simulink model "dual_ctrl_DWC"  (R2020b)
settings: Solver=VariableStepAuto  StartTime=0.0  StopTime=0.3  FixedStep=t_step
values from neighbouring files (symbols this model uses):
  a1 = 0.3    [Parameters_simulation_feb.m]
  a2 = 0.3    [Parameters_simulation_feb.m]
  b1 = 0.3    [Parameters_simulation_feb.m]
  b2 = 0.3    [Parameters_simulation_feb.m]
  C1 = 1/((w_opt^2)*L1)    [Parameters_simulation_feb.m]
  C2 = 1/((w_opt^2)*L2)    [Parameters_simulation_feb.m]
  h = 0.3    [Parameters_simulation_feb.m]
  L1 = (mu0/pi)*(N1^2)*(a1*log((2*a1*b1)/(r1*(a1+sqrt(a1^2 + b1^2)))) + b1*log((2*a1*b1)/(r1*(b1+sqrt(a1^2 + b1^2)))) - 2*(a1 +b1 - sqrt(a1^2 + b1^2)) + 0.25*(a1 + b1))    [Parameters_simulation_feb.m]
  L2 = (mu0/pi)*(N2^2)*(a2*log((2*a2*b2)/(r2*(a2+sqrt(a2^2 + b2^2)))) + b2*log((2*a2*b2)/(r2*(b2+sqrt(a2^2 + b2^2)))) - 2*(a2 +b2 - sqrt(a2^2 + b2^2)) + 0.25*(a2 + b2))    [Parameters_simulation_feb.m]
  M = (mu0/(4*pi))*N1*N2*(-M1 + M2 + M3 - M4)    [Parameters_simulation_feb.m]
  mu0 = 4*pi*1e-7    (= 1.25663706144e-06)    [Parameters_simulation_feb.m]
  N1 = N1_max    (= 2500)    [Parameters_simulation_feb.m]
  R1 = rho_cu*N1*2*(a1+b1)/S1    (= 51.6)    [Parameters_simulation_feb.m]
  R2 = rho_cu*N2*2*(a2+b2)/S2    (= 51.6)    [Parameters_simulation_feb.m]
  S1 = S1 + 2.5e-7    (= 1.25e-06)    [Parameters_simulation_feb.m]
  speed = 20    [Parameters_simulation_feb.m]
undefined symbols (not defined in the file or in its folder): Cb, Ion, k, ki_1, kp_1, Lb, Lithium, R, t_step, Vs
libraries: powerlib x61, eePowerMeasurement x6, powerlib_meascontrol x3, electricdrivelib x1, simulink x1
settings Model: Creator=Chuanyue Li  LastModifiedBy=c2107789
settings DataIOCC: ReturnWorkspaceOutputs=off
settings DebuggingCC: ArithmeticOperatorsInVariantConditions=warning
settings SFSimCC: SimUseLocalCustomCode=off  CustomCodeUndefinedFunction=UseInterfaceOnly
settings RTWCC: RTWUseLocalCustomCode=off

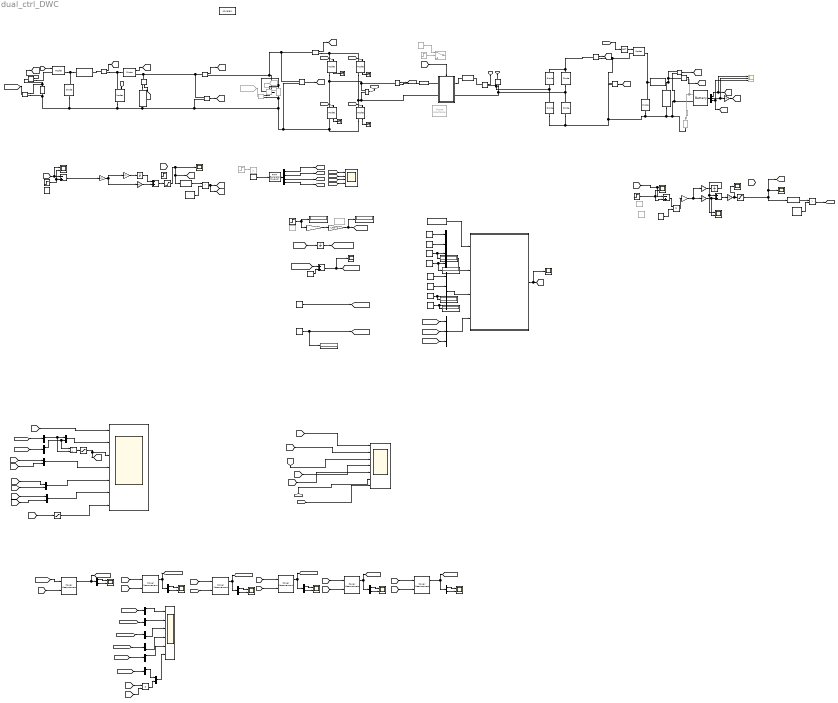
== system dual_ctrl_DWC ==
  note: Expanded implementation
  note: Inverter Control
  note: Buck-boost control
  note: Primary Coil
  note: Displacments & Airgap
  note: Velocity calc
  note: Assumed no vertical displacment
  note: Lateral (side) position
  note: Total distance moved from start
  note: assumed no side movement
  note: Height
  note: current position (relative to start)
  note: Mutual Inductance
  note: Position in driving direction
  note: Secondary Coil
  Add : Sum
  Add3 : Sum
  Add4 : Sum  Inputs=-+
  Add6 : Sum
  Add7 : Sum  Inputs=-+
  Battery1 : electricdrivelib/Extra Sources/Battery  BatType=Lithium-Ion  ShowTempParam=off  ThermalPreset=no  ShowAgeParam=off  NomV=400  NomQ=230  SOC=50  Batt_Tr=30  PresetModel=on  MaxQ=230  MinV=300  FullV=465.5949  Dis_rate=100  R=0.017391  Normal_OP=208  expZone="[432.1543          11.3]"  current=[6.5 13 32.5]  Units=Time  Tci=20  NomT=20  T2=-30  MaxQ2=4.8  FullV2=7.1  Normal_OP2=5.655  expZone2="[6.58           1]"  Rca=0.6  ti=2000  Dp=0  Neq0=0  Tsim=1e6  Ta1=25  Qeol=5.4*0.9  Reol=0.013333*1.2  Char_age=[2.3478, 3]  Dis_age=[2.3478, 10]  N1=1500  N2=10500  N3=1000  N4=1400  Ta2=45  N5=950
  Bus Creator{,1..3} (4 alike) : BusCreator  Inputs=2
  Bus Selector1 : BusSelector  OutputSignals=SOC (%),Current (A),Voltage (V)
  Constant : Constant  Value=0
  Constant1 : Constant  Value=h
  Constant2 : Constant  Value=40
  Constant3 : Constant  Commented=on  Value=10
  Constant4 : Constant
  Cp 1 : powerlib/Elements/Series RLC Branch  LConnTagsString=__new0  RConnTagsString=__new0  BranchType=C  Resistance=R  Inductance=1e-3  SetiL0=off  InitialCurrent=0  Capacitance=C1  Setx0=off  InitialVoltage=0  Measurements=None
  Cs 1 : powerlib/Elements/Series RLC Branch  LConnTagsString=__new0  RConnTagsString=__new0  BranchType=C  Resistance=R  Inductance=1e-3  SetiL0=off  InitialCurrent=0  Capacitance=C2  Setx0=off  InitialVoltage=0  Measurements=None
  Current Measurement{,1..3,7} (5 alike) : powerlib/Measurements/Current Measurement  PhasorSimulation=off  OutputType=Complex  PSBequivalent=0
  Current Measurement4 : powerlib/Measurements/Current Measurement  Commented=on  PhasorSimulation=off  OutputType=Complex  PSBequivalent=0
  DC Voltage Source : powerlib/Electrical Sources/DC Voltage Source  Amplitude=Vs  Measurements=None
  DC Voltage Source1 : powerlib/Electrical Sources/DC Voltage Source  Commented=on  Amplitude=Vs  Measurements=None
  DC Voltage Source2 : powerlib/Electrical Sources/DC Voltage Source  Commented=on  Amplitude=430  Measurements=None
  Demux : Demux
  Demux{1..14} (14 alike) : Demux  Outputs=2
  Diode : powerlib/Power Electronics/Diode  Ron=0.001  Lon=0  Vf=0  IC=0  UseSnubber=0  Rs=500000  Cs=250e-9  Measurements=on
  Diode1 : powerlib/Power Electronics/Diode  Ron=0.001  Lon=0  Vf=0.8  IC=0  UseSnubber=0  Rs=500  Cs=250e-9  Measurements=on
  Diode11 : powerlib/Power Electronics/Diode  Ron=0.001  Lon=0  Vf=0  IC=0  UseSnubber=0  Rs=500000  Cs=250e-9  Measurements=on
  Diode{2..4,7} (4 alike) : powerlib/Power Electronics/Diode  Ron=0.001  Lon=0  Vf=0.8  IC=0  UseSnubber=0  Rs=500  Cs=250e-9  Measurements=off
  Display{,1..3,5..7} (7 alike) : Display
  Divide : Product  Inputs=*/  OutMin=[0]  OutMax=[1]
  Fcn : Fcn  Expr=u(1)*2-1
  Fcn2 : Fcn  Expr=u(1)*2-1
  Gain : Gain  Gain=-1
  Gain10 : Gain  Gain=ki_1*10
  Gain11 : Gain  Gain=kp_1*10
  Gain12 : Gain  Gain=-1
  Gain13 : Gain  Gain=1e3
  Gain14 : Gain
  Gain5 : Gain  Gain=1/10
  Gain8 : Gain  Gain=k*0+1/100
  Goto18 : Goto  Commented=on  GotoTag=isource
  Goto26 : Goto  Commented=on  GotoTag=vsource
  I{2..3,8..9} (4 alike) : powerlib/Measurements/Current Measurement  PhasorSimulation=off  OutputType=Complex  PSBequivalent=0
  Initial_position : Constant  Value=-0.5
  Integrator : Integrator
  Integrator2 : Integrator  LimitOutput=on  UpperSaturationLimit=0  LowerSaturationLimit=-1
  Integrator3 : Integrator  InitialCondition=0.6
  MPH : Constant  Commented=on  Value=60
  Miles to m : Gain  Gain=1e3*1.609
  Mosfet : powerlib/Power Electronics/Mosfet  Ron=0.01  Lon=0  Rd=0.01  Vfd=0  IC=0  Rs=1e5  Cs=inf  Measurements=on
  Mosfet1 : powerlib/Power Electronics/Mosfet  Ron=0.01  Lon=0  Rd=0.01  Vfd=0  IC=0  Rs=1e5  Cs=inf  Measurements=on
  Mutual Inductance : powerlib/Elements/Mutual Inductance  Commented=on  LConnTagsString=a|b  RConnTagsString=A|B  TypeOfMutual=Two or three windings with equal mutual terms  NumberOfWindings=3  SelfImpedance1=[R1 L1]  SelfImpedance2=[R2 L2]  ThreeWindings=off  SelfImpedance3=[ 1.1 1.1e-03]  MutualImpedance=[0 M]  InductanceMatrix="[1.0 0.9  0.9 ;  0.9 1.0  0.9;  0.9 0.9 1.0 ] * 1e-3"  ResistanceMatrix="[1.0 0.9  0.9 ;  0.9 1.0  0.9;  0.9 0.9 1.0 ]"  Measurements=None
      settings: AttributesFormatString=\n  SourceProductBaseCode=PS
  Mutual_inductace_calculation : MATLAB Function  TreatAsAtomicUnit=on
  Mux : Mux  Inputs=2
  Mux1 : Mux
  Mux2 : Mux
  Mux3 : Mux  Inputs=3
  NOT : Logic  Operator=NOT  IconShape=distinctive  AllPortsSameDT=off  OutDataTypeStr=boolean
  N_primary2 : Constant  Value=N1
  N_secondary2 : Constant  Value=N1
  PWM Generator (2-Level)2 : powerlib_meascontrol/Pulse & Signal Generators/PWM Generator (2-Level)  ModulatorType=Single-phase full-bridge - Bipolar modulation (4 pulses)  ModulatorMode=Unsynchronized  Fc=f_opt  Pc=90  nF=27  MinMax="[ 0  1 ]"  SamplingTechnique=Natural  ModulatingSignals=off  m=0.8  Freq=60  Phase=0  Ts=0  ShowCarrierOutport=off
  Permiability2 : Constant  Value=mu0
  Power Measurement1 : eePowerMeasurement/Power Measurement  LabelModeActiveChoice=Continuous  F=20e3  K=[0 1]  Ts=0
      settings: SourceProductBaseCode=PS
  Power Measurement2 : eePowerMeasurement/Power Measurement  LabelModeActiveChoice=Continuous  F=s_fre  K=[0 1]  Ts=0
      settings: SourceProductBaseCode=PS
  Power Measurement{3..6} (4 alike) : eePowerMeasurement/Power Measurement  LabelModeActiveChoice=Continuous  F=f_opt  K=[0 1]  Ts=0
      settings: SourceProductBaseCode=PS
  Product : Product
  Product1 : Product  Commented=on
  Product2 : Product
  Ramp : simulink/Sources/Ramp  Commented=on  slope=200  start=0  InitialOutput=0
  Relational Operator : RelationalOperator  Operator=>  OutDataTypeStr=boolean  RndMeth=Zero
  Relational Operator2 : RelationalOperator  Operator=>  OutDataTypeStr=boolean  RndMeth=Zero
  S{3,9..12} (5 alike) : powerlib/Power Electronics/Mosfet  Ron=0.1  Lon=0  Rd=Rds  Vfd=0  IC=0  Rs=1e5  Cs=inf  Measurements=on
  S_primary2 : Constant  Value=S1
  S_secondary2 : Constant  Value=S1
  Saturation : Saturate  UpperLimit=inf  LowerLimit=0
  Saturation1 : Saturate  UpperLimit=0.95  LowerLimit=-1
  Saturation3 : Saturate  UpperLimit=1  LowerLimit=0
  Saturation4 : Saturate  UpperLimit=1  LowerLimit=0
  Scope : Scope  NumInputPorts=7
  Scope{1..2,4,19,22} (5 alike) : Scope
  Scope{6..10,12..13,18,21} (9 alike) : Scope  NumInputPorts=2
  Scope11 : Scope  NumInputPorts=4
  Scope14 : Scope  NumInputPorts=6
  Scope3 : Scope  NumInputPorts=7
  Scope5 : Scope  Commented=on  NumInputPorts=3
  Series RLC Branch : powerlib/Elements/Series RLC Branch  LConnTagsString=__new0  RConnTagsString=__new0  BranchType=L  Resistance=1  Inductance=Lb  SetiL0=on  InitialCurrent=100  Capacitance=1e-6  Setx0=off  InitialVoltage=0  Measurements=None
  Series RLC Branch1 : powerlib/Elements/Series RLC Branch  LConnTagsString=__new0  RConnTagsString=__new0  BranchType=C  Resistance=1  Inductance=1e-3  SetiL0=off  InitialCurrent=0  Capacitance=Cb  Setx0=on  InitialVoltage=400  Measurements=None
  Series RLC Branch3 : powerlib/Elements/Series RLC Branch  Commented=on  LConnTagsString=__new0  RConnTagsString=__new0  BranchType=R  Resistance=0.02  Inductance=1e-3  SetiL0=off  InitialCurrent=0  Capacitance=10e-3  Setx0=on  InitialVoltage=400  Measurements=None
  Series RLC Branch5 : powerlib/Elements/Series RLC Branch  LConnTagsString=__new0  RConnTagsString=__new0  BranchType=L  Resistance=1  Inductance=50e-3  SetiL0=on  InitialCurrent=10  Capacitance=1e-6  Setx0=off  InitialVoltage=0  Measurements=None
  Series RLC Branch9 : powerlib/Elements/Series RLC Branch  LConnTagsString=__new0  RConnTagsString=__new0  BranchType=C  Resistance=1  Inductance=1e-3  SetiL0=off  InitialCurrent=0  Capacitance=10e-3  Setx0=on  InitialVoltage=400  Measurements=None
  Step : Step  Commented=on  Time=0.05  Before=0.3  After=0.35  SampleTime=0
  Step1 : Step  Time=0  After=speed*0 + 10  SampleTime=0
  Step19 : Step  Time=0.1  Before=10  After=12  SampleTime=0
  Step2 : Step  Time=0.3  Before=0.5  After=0.5  SampleTime=0
  Step3 : Step  Commented=on  Time=0.02  Before=1  After=0  SampleTime=0
  Step4 : Step  Time=0.05  Before=100  After=50  SampleTime=0
  Subsystem1 : Subsystem
      settings: PortSchema="{\"entries\":[{\"content\":{\"sides\":[{\"content\":{\"connectorIds\":[\"LConn1\",\"LConn2\"]},\"type\":\"ConnectorPlacement.EquallySpacedRectSide\",\"uuid\":\"dc2bcdb6-339b-4429-bac0-92f3c92c18cf\"},{\"content\":{\"connectorIds\":[\"RConn1\",\"RConn2\"],\"side\":\"RIGHT\"},\"type\":\"ConnectorPlacement.EquallySpacedRectSide\",\"uuid\":\"b0ad11da-e286-4d85-af23-59a8fde2f407\"},{\"content\":{\"connectorIds\":[\"In1\"],\"side\":\"TOP\"},\"type\":\"ConnectorPlacement.EquallySpacedRectSide\",\"uuid\":\"877cda52-a106-40c9-ba33-8eb6041f6ad7\"},{\"content\":{\"connectorIds\":[],\"side\":\"HIDDEN\"},\"type\":\"ConnectorPlacement.EquallySpacedRectSide\",\"uuid\":\"0e4f87e0-ec1d-4257-a5bd-1d06479f0226\"}]},\"type\":\"ConnectorPlacement.EquallySpacedConnector\",\"uuid\":\"a87b5a18-e0dc-451c-be30-4cd433b35579\"}],\"packageUris\":[\"http://schema.mathworks.com/mf0/Connector/R2020b\"],\"version\":\"1.0\"}"
  Switch : Switch  Commented=on  Criteria=u2 > Threshold
  Terminator{16..17,22..23} (4 alike) : Terminator
  Triangle Generator : powerlib_meascontrol/Pulse & Signal Generators/Triangle Generator  Freq=s_fre  Phase=0  Ts=0
  Triangle Generator2 : powerlib_meascontrol/Pulse & Signal Generators/Triangle Generator  Freq=s_fre  Phase=0  Ts=0
  V_S1 : powerlib/Measurements/Voltage Measurement  PhasorSimulation=off  OutputType=Complex  PSBequivalent=0
  V_S2 : powerlib/Measurements/Voltage Measurement  PhasorSimulation=off  OutputType=Complex  PSBequivalent=0
  V_S3 : powerlib/Measurements/Voltage Measurement  PhasorSimulation=off  OutputType=Complex  PSBequivalent=0
  V_p2 : powerlib/Measurements/Voltage Measurement  PhasorSimulation=off  OutputType=Complex  PSBequivalent=0
  Voltage Measurement : powerlib/Measurements/Voltage Measurement  PhasorSimulation=off  OutputType=Complex  PSBequivalent=0
  Voltage Measurement1 : powerlib/Measurements/Voltage Measurement  Commented=on  PhasorSimulation=off  OutputType=Complex  PSBequivalent=0
  Voltage Measurement2 : powerlib/Measurements/Voltage Measurement  PhasorSimulation=off  OutputType=Complex  PSBequivalent=0
  Voltage Measurement5 : powerlib/Measurements/Voltage Measurement  PhasorSimulation=off  OutputType=Complex  PSBequivalent=0
  Zero : Constant  Commented=on  Value=0  OutDataTypeStr=Inherit: Inherit via back propagation
  Zero1 : Constant  Value=0.5  OutDataTypeStr=Inherit: Inherit via back propagation
  a_primary1 : Constant  Value=a1
  a_secondary2 : Constant  Value=a2
  b_primary2 : Constant  Value=b1
  b_secondary2 : Constant  Value=b2
  hour to seconds : Gain  Gain=1/60^2
  ms-1 : Constant  Commented=on  Value=speed
  powergui : powerlib/powergui  Priority=1  SimulationMode=Continuous  SampleTime=t_step  frequency=60  Iterations=50  frequencyindice=0  Pbase=100e6  ErrMax=1e-4  UnitsV=kV  UnitsW=MW  buscounter=0  FunctionMessages=off  echomessages=off  EnableUseOfTLC=off  CurrentSourceSwitches=off  DisableSnubberDevices=off  DisableRonSwitches=off  DisableVfSwitches=off  DisplayEquations=off  AutomaticDiscreteSolvers=off  SolverType=Tustin/Backward Euler (TBE)  Interpol=off  ExternalGateDelay=off  methode=off  Ts=100  x0status=blocks  SPID=off  SwTol=0  HookPort=off  NonlinearTolerance=1e-4  nMaxIteration=100  ContinueOnMaxIteration=off  RestoreLinks=warning  ResistiveCurrentMeasurement=off  Frange=[0:2:500]  Ylog=off  Xlog=on  ShowGrid=off  save=off  variable=ZData  structure=logsout  ZoomFFT=off  StartTime=0.2  cycles=10  DisplayStyle=2  fundamental=50  FreqAxis=off  MaxFrequency=1000  frequencyindicesteady=1  RmsSteady=1  display=off
  wires:
  Demux/4 -> [S4]
  [S3] -> Scope11/3
  Demux/3 -> [S3]
  [S4] -> S10/1
  I8/1 -> [Ip1]
  Demux/1 -> [S1]
  [S2] -> Scope11/2
  S12/1 -> Terminator17/1
  S11/1 -> Terminator23/1
  [S4] -> Scope11/4
  S10/1 -> Terminator16/1
  Current Measurement3/1 -> [I_in]  "Input Current"
  [S2] -> S12/1
  S9/1 -> Terminator22/1
  [S3] -> S11/1
  V_p2/1 -> [V_p1]
  [S1] -> Scope11/1
  PWM Generator (2-Level)2/1 -> Demux/1
  Demux/2 -> [S2]
  V_S2/1 -> [Vs1]  "v2"
  Step/1 -> Product1/1
  [S1] -> S9/1
  I9/1 -> [Is1]  "i2"
  Zero1/1 -> PWM Generator (2-Level)2/1
  Integrator3/1 -> Add6/1
  Fcn/1 -> Relational Operator/1
  Add6/1 -> Saturation1/1
  Diode11/1 -> [iDIO]
  [s2] -> Mosfet1/1
  Current Measurement/1 -> [il]
  Current Measurement1/1 -> [io_dcdc]
  Gain10/1 -> Integrator3/1
  Current Measurement2/1 -> [ic]
  Triangle Generator/1 -> Relational Operator/2
  [s1] -> Mosfet/1
  Add7/1 -> Gain8/1
  [il] -> Scope7/1, Add7/1
  Gain8/1 -> Gain11/1, Gain10/1
  Voltage Measurement/1 -> [vc]
  Relational Operator/1 -> [s1], [s2]
  Step4/1 -> Scope7/2, Add7/2  "il_target"
  Gain11/1 -> Add6/2
  Current Measurement7/1 -> [isource]
  [isource] -> Power Measurement1/2
  Voltage Measurement5/1 -> [vsource]
  [vsource] -> Power Measurement1/1
  Power Measurement1/1 -> [input_power], Demux3/1  "Input power (source)"
  Demux3/2 -> Scope18/2
  Demux3/1 -> Scope18/1
  Gain13/1 -> Integrator2/1
  Gain5/1 -> Gain13/1, Gain14/1
  Product/1 -> Gain5/1
  Battery1/1 -> Bus Selector1/1
  Saturation4/1 -> [d_REC], Scope22/1, Fcn2/1
  Integrator2/1 -> Scope8/1, Add3/1
  Gain14/1 -> Scope8/2, Add3/2
  Bus Selector1/1 -> Scope5/1, [SOC]  "<SOC (%)>"
  Bus Selector1/3 -> [Vo_b], Scope5/3  "<Voltage (V)>"
  Gain/1 -> [Io_b]
  Fcn2/1 -> Relational Operator2/1
  Triangle Generator2/1 -> Relational Operator2/2
  Gain12/1 -> Scope19/1, Saturation4/1
  Add3/1 -> Gain12/1
  Relational Operator2/1 -> [t1]
  Step19/1 -> Add4/2, Scope21/2  "io_target"
  Bus Selector1/2 -> Scope5/2, Gain/1  "<Current (A)>"
  Saturation1/1 -> Fcn/1, [D], Scope4/1  "D1"
  [input_power] -> Demux1/1
  Bus Creator/1 -> Scope3/2  "power_comp"
  [Vo] -> Power Measurement2/1
  [Io] -> Power Measurement2/2
  Demux2/1 -> Scope6/1
  Demux2/2 -> Scope6/2
  Power Measurement2/1 -> Demux2/1, [output_power]
  [output_power] -> Demux4/1
  Demux1/1 -> Bus Creator/1, Divide/2  "input power"
  Demux4/1 -> Bus Creator/2, Divide/1  "output power"
  Saturation3/1 -> [eff], Scope3/3  "efficiency"
  Divide/1 -> Saturation3/1  "efficiency"
  [D] -> Bus Creator1/1  "praimry buck bost"
  [d_REC] -> Bus Creator1/2  "secondary rectifier"
  V_S1/1 -> [vrec]  "vrrec"
  [il] -> Bus Creator2/1  "praimry buck boost"
  [irec] -> Bus Creator2/2  "secondary rectifier output"
  Bus Creator2/1 -> Scope3/5  "inductor currents"
  [vc] -> Bus Creator3/1  "primary buck boost"
  [vrec] -> Bus Creator3/2  "secondary rectifier output"
  Bus Creator3/1 -> Scope3/6  "capcitor voltages"
  Bus Creator1/1 -> Scope3/4  "duty cycles"
  [Io] -> Saturation/1  "output current"
  [eff] -> Scope/1  "eff"
  [il] -> Scope/2  "il"
  [ic] -> Scope/3  "ic"
  [vc] -> Scope/4  "vc"
  [io_dcdc] -> Scope/5  "iodc"
  [V_p1] -> Scope/6  "vp"
  [Ip1] -> Scope/7  "Ip"
  a_primary1/1 -> Display/1, Mux1/3  "width (x)"
  Mutual_inductace_calculation/1(M) -> [M], Scope2/1
  Integrator/1 -> [displacment]
  hour to seconds/1 -> Display7/1, [speed_ms]
  Mux3/1 -> Mutual_inductace_calculation/4(displacments)
  [speed_ms] -> Integrator/1  "speed"
  Constant/1 -> [side_position]
  Step1/1 -> Display6/1, Miles to m/1
  Miles to m/1 -> hour to seconds/1
  [displacment] -> Add/1
  Mux1/1 -> Mutual_inductace_calculation/2(params_primary)  "Primary coil parameters"
  [side_position] -> Mux3/1  "x"
  S_secondary2/1 -> Mux2/2
  b_secondary2/1 -> Display3/1, Mux2/4  "height (y)"
  N_primary2/1 -> Mux1/1
  Mux2/1 -> Mutual_inductace_calculation/3(params_secondary)  "Secondary Coil Parameters"
  S_primary2/1 -> Mux1/2
  N_secondary2/1 -> Mux2/1
  [height_position] -> Mux3/3  "airgap"
  Permiability2/1 -> Mutual_inductace_calculation/1(mu)
  Add/1 -> Scope1/1, [fwd_position]  "position"
  [fwd_position] -> Mux3/2  "y"
  Initial_position/1 -> Add/2
  b_primary2/1 -> Display1/1, Mux1/4  "height (y)"
  Constant1/1 -> Display5/1, [height_position]
  a_secondary2/1 -> Display2/1, Mux2/3  "width (x)"
  Zero/1 -> Switch/1  "M"
  Step3/1 -> Switch/2
  [M] -> Subsystem1/1(M)  "M"
  [M] -> Scope3/1  "Mutual Inductance"
  Current Measurement4/1 -> Goto18/1
  Voltage Measurement1/1 -> Goto26/1
  Add4/1 -> Product/1
  Constant4/1 -> Product/2
  V_S3/1 -> [Vo]  "vcap"
  Saturation/1 -> Scope3/7  "Output Current"
  [t1] -> NOT/1
  NOT/1 -> S3/1
  I2/1 -> [Io]
  [Io] -> Add4/1, Scope21/1
  I3/1 -> [irec]
  [vrec] -> Power Measurement3/1
  [irec] -> Power Measurement3/2
  Power Measurement3/1 -> [rectifier_power], Demux5/1
  Demux5/2 -> Scope9/2
  Demux5/1 -> Scope9/1
  Demux6/1 -> Scope10/1
  Demux6/2 -> Scope10/2
  Power Measurement4/1 -> Demux6/1, [secondary_power]
  [Is1] -> Power Measurement4/2
  [Vs1] -> Power Measurement4/1
  [V_p1] -> Power Measurement5/1
  [Ip1] -> Power Measurement5/2
  Power Measurement5/1 -> [primary_power], Demux7/1
  Demux7/2 -> Scope12/2
  Demux7/1 -> Scope12/1
  Voltage Measurement2/1 -> [V_in]
  Demux8/1 -> Scope13/1
  Demux8/2 -> Scope13/2
  Power Measurement6/1 -> Demux8/1, [inv_input_power]
  [I_in] -> Power Measurement6/2
  [V_in] -> Power Measurement6/1
  [input_power] -> Demux9/1
  Demux9/1 -> Scope14/1
  [inv_input_power] -> Demux10/1
  Demux10/1 -> Scope14/2
  [primary_power] -> Demux11/1
  Demux11/2 -> Scope14/3
  Demux12/2 -> Scope14/4
  [secondary_power] -> Demux12/1
  Demux13/1 -> Scope14/5
  [rectifier_power] -> Demux13/1
  [output_power] -> Demux14/1
  Demux14/1 -> Mux/1
  Mux/1 -> Scope14/6
  Product2/1 -> Mux/2
  [Vo] -> Product2/1
  [Io] -> Product2/2
  connections:
  DC Voltage Source1/LConn1 -- Voltage Measurement1/LConn2 -- Voltage Measurement2/LConn2 -- S10/RConn1 -- S12/RConn1 -- Diode/LConn1 -- Voltage Measurement5/LConn2 -- DC Voltage Source/LConn1 -- Mosfet1/RConn1 -- Series RLC Branch1/RConn1 -- Voltage Measurement/LConn2
  V_p2/LConn2 -- Subsystem1/LConn2 -- S11/RConn1 -- S10/LConn1
  V_S2/LConn1 -- I9/RConn1 -- Diode7/RConn1 -- Diode2/LConn1
  Current Measurement3/RConn1 -- S11/LConn1 -- S9/LConn1
  V_p2/LConn1 -- S9/RConn1 -- S12/LConn1 -- I8/LConn1
  V_S2/LConn2 -- Subsystem1/RConn2 -- Diode3/RConn1 -- Diode4/LConn1
  I8/RConn1 -- Cp 1/RConn1
  Subsystem1/RConn1 -- Cs 1/LConn1
  I9/LConn1 -- Cs 1/RConn1
  Subsystem1/LConn1 -- Cp 1/LConn1
  Current Measurement3/LConn1 -- Voltage Measurement2/LConn1 -- Current Measurement4/RConn1 -- Current Measurement1/RConn1
  Series RLC Branch/LConn1 -- Mosfet/RConn1 -- Diode/RConn1
  Diode11/LConn1 -- Mosfet1/LConn1 -- Current Measurement/RConn1
  Diode11/RConn1 -- Current Measurement1/LConn1 -- Voltage Measurement/LConn1 -- Current Measurement2/LConn1
  Current Measurement/LConn1 -- Series RLC Branch/RConn1
  Current Measurement7/RConn1 -- Mosfet/LConn1
  Current Measurement2/RConn1 -- Series RLC Branch1/LConn1
  Battery1/LConn2 -- V_S3/LConn2 -- DC Voltage Source2/LConn1 -- Series RLC Branch9/RConn1 -- Diode3/LConn1 -- Diode7/LConn1 -- V_S1/LConn2 -- Diode1/LConn1
  Current Measurement7/LConn1 -- Voltage Measurement5/LConn1 -- DC Voltage Source/RConn1
  Series RLC Branch5/LConn1 -- S3/RConn1 -- Diode1/RConn1
  DC Voltage Source1/RConn1 -- Current Measurement4/LConn1 -- Voltage Measurement1/LConn1
  V_S1/LConn1 -- I3/RConn1 -- S3/LConn1
  Series RLC Branch9/LConn1 -- I2/LConn1 -- V_S3/LConn1 -- Series RLC Branch5/RConn1
  DC Voltage Source2/RConn1 -- Series RLC Branch3/RConn1
  Series RLC Branch3/LConn1 -- I2/RConn1 -- Battery1/LConn1
  I3/LConn1 -- Diode2/RConn1 -- Diode4/RConn1

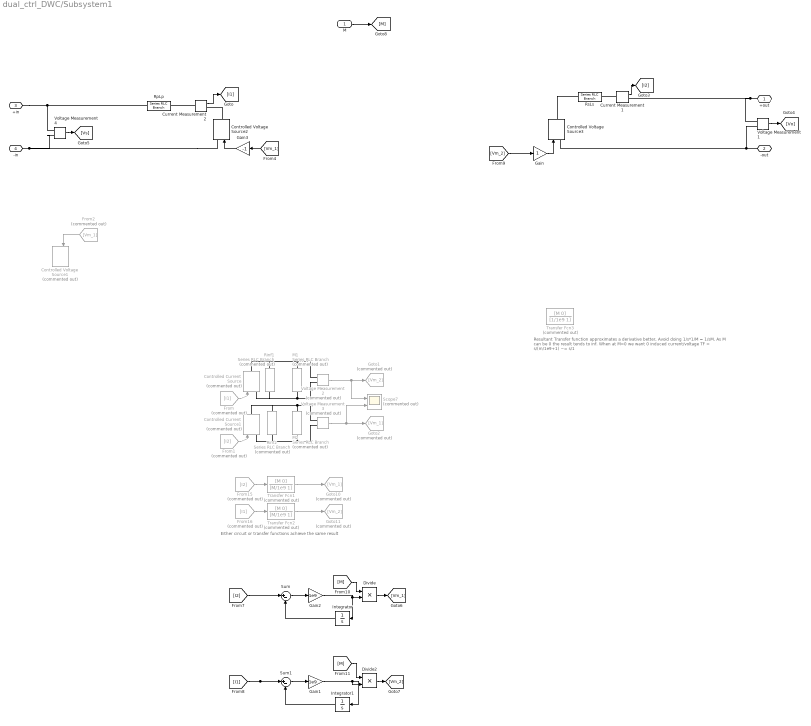
== system dual_ctrl_DWC/Subsystem1 ==
  note: Resultant Transfer function approximates a derivative better,
      | Avoid doing 1/s*1/M = 1/sM. As M can be 0 the result tends to inf. When at M=0 we want 0 induced current/voltage
      |
      | TF = s/(m/1e9+1) ~= s/1
  note: Either circuit or transfer functions achieve the same result
  M : Inport
  Controlled Current Source : powerlib/Electrical Sources/Controlled Current Source  Commented=on  Initialize=on  Source_Type=AC  Amplitude=0  Phase=0  Frequency=0  Measurements=None
  Controlled Current Source1 : powerlib/Electrical Sources/Controlled Current Source  Commented=on  Initialize=on  Source_Type=AC  Amplitude=0  Phase=0  Frequency=0  Measurements=None
  Controlled Voltage Source1 : powerlib/Electrical Sources/Controlled Voltage Source  Commented=on  Initialize=on  Source_Type=AC  Amplitude=0  Phase=0  Frequency=0  Measurements=None
  Controlled Voltage Source2 : powerlib/Electrical Sources/Controlled Voltage Source  Initialize=on  Source_Type=AC  Amplitude=0  Phase=0  Frequency=0  Measurements=None
  Controlled Voltage Source3 : powerlib/Electrical Sources/Controlled Voltage Source  Initialize=on  Source_Type=AC  Amplitude=0  Phase=0  Frequency=0  Measurements=None
  Current Measurement1 : powerlib/Measurements/Current Measurement  PhasorSimulation=off  OutputType=Complex  PSBequivalent=0
  Current Measurement2 : powerlib/Measurements/Current Measurement  PhasorSimulation=off  OutputType=Complex  PSBequivalent=0
  Divide : Product  Inputs=**
  Divide2 : Product  Inputs=**
  From : From  Commented=on  GotoTag=I1
  From1 : From  Commented=on  GotoTag=I2
  From15 : From  Commented=on  GotoTag=I2
  From16 : From  Commented=on  GotoTag=I1
  From2 : From  Commented=on  GotoTag=Vm_1
  Gain : Gain
  Gain1 : Gain  Gain=1e9
  Gain2 : Gain  Gain=1e9
  Gain3 : Gain  Gain=-1
  Goto1 : Goto  Commented=on  GotoTag=Vm_2
  Goto10 : Goto  Commented=on  GotoTag=Vm_1
  Goto11 : Goto  Commented=on  GotoTag=Vm_2
  Goto2 : Goto  Commented=on  GotoTag=Vm_1
  Integrator : Integrator
  Integrator1 : Integrator
  M1 : powerlib/Elements/Series RLC Branch  Commented=on  LConnTagsString=__new0  RConnTagsString=__new0  BranchType=L  Resistance=R  Inductance=M  SetiL0=off  InitialCurrent=0  Capacitance=C1  Setx0=off  InitialVoltage=0  Measurements=None
  "M2 " : powerlib/Elements/Series RLC Branch  Commented=on  LConnTagsString=__new0  RConnTagsString=__new0  BranchType=L  Resistance=R  Inductance=M  SetiL0=off  InitialCurrent=0  Capacitance=C1  Setx0=off  InitialVoltage=0  Measurements=None
  Rinf1 : powerlib/Elements/Series RLC Branch  Commented=on  LConnTagsString=__new0  RConnTagsString=__new0  BranchType=R  Resistance=1e9  Inductance=M  SetiL0=off  InitialCurrent=0  Capacitance=C1  Setx0=off  InitialVoltage=0  Measurements=None
  "Rinf2 " : powerlib/Elements/Series RLC Branch  Commented=on  LConnTagsString=__new0  RConnTagsString=__new0  BranchType=R  Resistance=1e9  Inductance=M  SetiL0=off  InitialCurrent=0  Capacitance=C1  Setx0=off  InitialVoltage=0  Measurements=None
  RpLp : powerlib/Elements/Series RLC Branch  LConnTagsString=__new0  RConnTagsString=__new0  BranchType=RL  Resistance=R1  Inductance=L1  SetiL0=off  InitialCurrent=0  Capacitance=C1  Setx0=off  InitialVoltage=0  Measurements=None
  RsLs : powerlib/Elements/Series RLC Branch  LConnTagsString=__new0  RConnTagsString=__new0  BranchType=RL  Resistance=R2  Inductance=L2  SetiL0=off  InitialCurrent=0  Capacitance=C1  Setx0=off  InitialVoltage=0  Measurements=None
  Scope7 : Scope  Commented=on  NumInputPorts=2
  Sum : Sum  Inputs=|+-
  Sum1 : Sum  Inputs=|+-
  Transfer Fcn1 : TransferFcn  Commented=on  Numerator=[M 0]  Denominator=[M/1e9 1]
  Transfer Fcn2 : TransferFcn  Commented=on  Numerator=[M 0]  Denominator=[M/1e9 1]
  Transfer Fcn3 : TransferFcn  Commented=on  Numerator=[M 0]  Denominator=[1/1e9 1]
  Voltage Measurement1 : powerlib/Measurements/Voltage Measurement  PhasorSimulation=off  OutputType=Complex  PSBequivalent=0
  Voltage Measurement2 : powerlib/Measurements/Voltage Measurement  Commented=on  PhasorSimulation=off  OutputType=Complex  PSBequivalent=0
  Voltage Measurement3 : powerlib/Measurements/Voltage Measurement  Commented=on  PhasorSimulation=off  OutputType=Complex  PSBequivalent=0
  Voltage Measurement4 : powerlib/Measurements/Voltage Measurement  PhasorSimulation=off  OutputType=Complex  PSBequivalent=0
  +out : PMIOPort  Side=Right
  -out : PMIOPort  Port=2  Side=Right
  +in : PMIOPort  Port=3  Side=Left
  -in : PMIOPort  Port=4  Side=Left
  wires:
  [M] -> Divide2/1
  Divide2/1 -> [Vm_2]
  [M] -> Divide/1
  Divide/1 -> [Vm_1]
  M/1 -> [M]
  Gain1/1 -> Divide2/2, Integrator1/1
  Gain2/1 -> Divide/2, Integrator/1
  [I1] -> Sum1/1
  Sum1/1 -> Gain1/1
  Integrator1/1 -> Sum1/2
  Integrator/1 -> Sum/2
  Sum/1 -> Gain2/1
  [I2] -> Sum/1
  From16/1 -> Transfer Fcn2/1
  Transfer Fcn1/1 -> Goto10/1
  From15/1 -> Transfer Fcn1/1
  Transfer Fcn2/1 -> Goto11/1
  Voltage Measurement4/1 -> [Vs]
  Voltage Measurement1/1 -> [Vo]
  Gain/1 -> Controlled Voltage Source3/1
  Voltage Measurement2/1 -> Scope7/1, Goto1/1
  Voltage Measurement3/1 -> Scope7/2, Goto2/1
  Current Measurement2/1 -> [I1]
  From/1 -> Controlled Current Source/1
  Current Measurement1/1 -> [I2]
  From1/1 -> Controlled Current Source1/1
  [Vm_2] -> Gain/1
  [Vm_1] -> Gain3/1
  From2/1 -> Controlled Voltage Source1/1
  Gain3/1 -> Controlled Voltage Source2/1
  connections:
  "M2 "/LConn1 -- Voltage Measurement3/LConn2 -- "Rinf2 "/LConn1 -- Controlled Current Source1/LConn1
  "M2 "/RConn1 -- Voltage Measurement3/LConn1 -- Controlled Current Source1/RConn1 -- "Rinf2 "/RConn1
  Controlled Voltage Source3/RConn1 -- RsLs/LConn1
  M1/LConn1 -- Controlled Current Source/LConn1 -- Rinf1/LConn1 -- Voltage Measurement2/LConn2
  M1/RConn1 -- Voltage Measurement2/LConn1 -- Rinf1/RConn1 -- Controlled Current Source/RConn1
  Voltage Measurement1/LConn2 -- Controlled Voltage Source3/LConn1 -- -out/RConn1
  -in/RConn1 -- Controlled Voltage Source2/LConn1 -- Voltage Measurement4/LConn2
  Controlled Voltage Source2/RConn1 -- Current Measurement2/RConn1
  +out/RConn1 -- Voltage Measurement1/LConn1 -- Current Measurement1/RConn1
  +in/RConn1 -- Voltage Measurement4/LConn1 -- RpLp/LConn1
  Current Measurement1/LConn1 -- RsLs/RConn1
  Current Measurement2/LConn1 -- RpLp/RConn1

== matlab function dual_ctrl_DWC/Mutual_inductace_calculation ==
  data: mu input; M output; params_primary input; params_secondary input; displacments input
function M = M_calc(mu, params_primary, params_secondary, displacments)


mu0 = mu; %permeability of free space 

%% transmitter coil
N1 = params_primary(1); % Number of primary turns
S1 = params_primary(2); % Number of primary winding sections
a1 = params_primary(3); % Width of primary winding
b1 = params_primary(4); % Length of primary winding

%% receiver coil
N2 = params_secondary(1); % Number of reciever turns
S2 = params_secondary(2); % Number of secondary winding sections
a2 = params_secondary(3); % Width of secondary winding
b2 = params_secondary(4); % Width of secondary winding

%% Distances
c = displacments(1);
e = displacments(2);
h = displacments(3);

d = a1 -a2 - c;
m = a2 + c;
q = b2 + e;
g = a1 - c;
p = b1 - e;
t = b1 - b2 - e;

%% Mutual inductance
M1_ = ((d*log((d+sqrt(h^2 + (-t)^2 + d^2))/(d + sqrt(h^2 + d^2 + q^2)))) + (g*log((g+sqrt(h^2 + (q)^2 + g^2))/(g + sqrt(h^2 + g^2 + (-t)^2)))) + (c*log(((-c)+sqrt(h^2 + (q)^2 + c^2))/((-c) + sqrt(h^2 + c^2 + (-t)^2)))) + (m*log(((-m)+sqrt(h^2 + (-t)^2 + m^2))/((-m) + sqrt(h^2 + m^2 + q^2)))) + sqrt(h^2 + q^2 + d^2) - sqrt(h^2 + q^2 + g^2) - sqrt(h^2 + q^2 + m^2) + sqrt(h^2 + q^2 + c^2) + sqrt(h^2 + (-t)^2 + g^2) - sqrt(h^2 + (-t)^2 + d^2) + sqrt(h^2 + (-t)^2 + m^2) - sqrt(h^2 + (-t)^2 + c^2));
M2_ = ((d*log((d+sqrt(h^2 + (-p)^2 + d^2))/(d + sqrt(h^2 + d^2 + e^2)))) + (g*log((g+sqrt(h^2 + (e)^2 + g^2))/(g + sqrt(h^2 + g^2 + (-p)^2)))) + (c*log(((-c)+sqrt(h^2 + (e)^2 + c^2))/((-c) + sqrt(h^2 + c^2 + (-p)^2)))) + (m*log(((-m)+sqrt(h^2 + (-p)^2 + m^2))/((-m) + sqrt(h^2 + m^2 + e^2)))) + sqrt(h^2 + e^2 + d^2) - sqrt(h^2 + e^2 + g^2) - sqrt(h^2 + e^2 + m^2) + sqrt(h^2 + e^2 + c^2) + sqrt(h^2 + (-p)^2 + g^2) - sqrt(h^2 + (-p)^2 + d^2) + sqrt(h^2 + (-p)^2 + m^2) - sqrt(h^2 + (-p)^2 + c^2));
M3_ = ((t*log((t+sqrt(h^2 + (-g)^2 + t^2))/(t + sqrt(h^2 + t^2 + c^2)))) + (p*log((p+sqrt(h^2 + (p)^2 + c^2))/(p + sqrt(h^2 + (-g)^2 + p^2)))) + (e*log(((-e)+sqrt(h^2 + (e)^2 + c^2))/((-e) + sqrt(h^2 + e^2 + (-g)^2)))) + (q*log(((-q)+sqrt(h^2 + (-g)^2 + q^2))/((-q) + sqrt(h^2 + c^2 + q^2)))) + sqrt(h^2 + c^2 + t^2) - sqrt(h^2 + c^2 + p^2) - sqrt(h^2 + c^2 + q^2) + sqrt(h^2 + e^2 + c^2) + sqrt(h^2 + (-g)^2 + p^2) - sqrt(h^2 + (-g)^2 + t^2) + sqrt(h^2 + (-g)^2 + q^2) - sqrt(h^2 + (-g)^2 + e^2));
M4_ = ((t*log((t+sqrt(h^2 + (-d)^2 + t^2))/(t + sqrt(h^2 + t^2 + m^2)))) + (p*log((p+sqrt(h^2 + (m)^2 + p^2))/(p + sqrt(h^2 + (-d)^2 + p^2)))) + (e*log(((-e)+sqrt(h^2 + (e)^2 + m^2))/((-e) + sqrt(h^2 + e^2 + (-d)^2)))) + (q*log(((-q)+sqrt(h^2 + (-d)^2 + q^2))/((-q) + sqrt(h^2 + m^2 + q^2)))) + sqrt(h^2 + m^2 + t^2) - sqrt(h^2 + m^2 + p^2) - sqrt(h^2 + m^2 + q^2) + sqrt(h^2 + e^2 + m^2) + sqrt(h^2 + (-d)^2 + p^2) - sqrt(h^2 + (-d)^2 + t^2) + sqrt(h^2 + (-d)^2 + q^2) - sqrt(h^2 + (-d)^2 + e^2)); 
M = (mu0/(4*pi))*N1*N2*(-M1_ + M2_ + M3_ - M4_); %Appears to be correct
% M = (mu0/(4*pi))*N1*N2*(M1_ - M2_ + M3_ - M4_); %As shown in literature
